simulink model "sv_model"  (R2012b)
settings: Solver=ode45  StartTime=0.0  StopTime=Tf  MaxStep=1e-3  RelTol=1e-3
values from neighbouring files (symbols this model uses):
  A = [0 1; -2 -3]    [sv__feedback__observer_driver.m]    (also in sv__feedback__observer_type1_driver.m; sv__feedback_driver.m; sv__feedback_type1_driver.m; tf_sv_driver.m)
  B = [1; 0]    [sv__feedback__observer_driver.m]    (also in sv__feedback__observer_type1_driver.m; sv__feedback_driver.m; sv__feedback_type1_driver.m; tf_sv_driver.m)
  C = [1 0]    [sv__feedback__observer_driver.m]    (also in sv__feedback__observer_type1_driver.m = [0 1]; sv__feedback_driver.m; sv__feedback_type1_driver.m; tf_sv_driver.m)
  den_Gpre = C_obs*inv(A_obs-B_obs*K)*B_obs    [sv__feedback__observer_driver.m]    (also in sv__feedback_driver.m = C*inv(A-B*K)*B; tf_sv_driver.m = 1)
  num_Gpre = -1    [sv__feedback__observer_driver.m]    (also in sv__feedback_driver.m; tf_sv_driver.m = 1)
undefined symbols (not defined in the file or in its folder): den_Gc, num_Gc
settings Model: Creator=student  LastModifiedBy=throne
settings DataIOCC: SignalLoggingSaveFormat=ModelDataLogs  SignalLoggingName=sigsOut
settings OptimizationCC: InitFltsAndDblsToZero=on
settings DebuggingCC: SaveWithParameterizedLinksMsg=none  SignalResolutionControl=TryResolveAllWithWarning  SolverPrmCheckMsg=none  MultiTaskDSMMsg=warning  MultiTaskCondExecSysMsg=none  FcnCallInpInsideContextMsg=UseLocalSettings  StrictBusMsg=None
settings HardwareCC: TargetUnknown=on
settings RTWCC: IncludeERTFirstTime=on
settings GRTTargetCC: CombineOutputUpdateFcns=off  GRTInterface=on

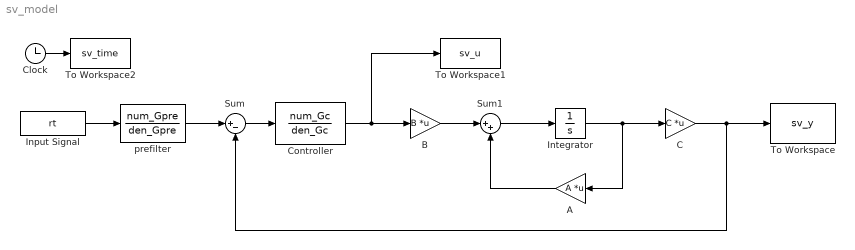
== system sv_model ==
  A : Gain  Gain=A  Multiplication=Matrix(K*u)
  B : Gain  Gain=B  Multiplication=Matrix(K*u)
  C : Gain  Gain=C  Multiplication=Matrix(K*u)
  Clock : Clock
  Controller : TransferFcn  Numerator=num_Gc  Denominator=den_Gc
  "Input Signal " : FromWorkspace  VariableName=rt  SampleTime=0
  Integrator : Integrator
  Sum : Sum  Inputs=|+-  SaturateOnIntegerOverflow=on
  Sum1 : Sum  Inputs=|++
  To Workspace : ToWorkspace  VariableName=sv_y  SampleTime=-1
  To Workspace1 : ToWorkspace  VariableName=sv_u  SampleTime=-1
  To Workspace2 : ToWorkspace  VariableName=sv_time  SampleTime=-1
  prefilter : TransferFcn  Numerator=num_Gpre  Denominator=den_Gpre
  wires:
  Sum/1 -> Controller/1
  Clock/1 -> To Workspace2/1
  prefilter/1 -> Sum/1
  "Input Signal "/1 -> prefilter/1
  Controller/1 -> B/1, To Workspace1/1
  B/1 -> Sum1/1
  Sum1/1 -> Integrator/1
  Integrator/1 -> A/1, C/1
  A/1 -> Sum1/2
  C/1 -> Sum/2, To Workspace/1
